simulink model "IEEE34bus_v2019b_Phasor_PI"  (R2019b)
settings: Solver=ode4  StartTime=0.0  StopTime=100  FixedStep=Ts  MaxStep=1e-4  RelTol=1e-4
InitFcn:
  | a=1; % Loading Factor
  | Ts=0.1;% For Delay Blocks in Voltage Regulator Controls
  | % phase to sequence conversion of RXB matrices
  | c=1*exp(sqrt(-1)*(120*pi/180));
  | T=[1 1 1;1 c*c c;1 c c*c];
  | Tinv=1/3*[1 1 1;1 c c*c;1 c*c c];
  | 
  | % Simulation data for the IEEE 34 Node Test Feeder model
  | mi2km = 1.60934;%  miles to km conversion
  | ft2km = 0.0003048; % feet to km conversion
  | ms2F = 1*1e-6/(2*pi*60);% microsiemens to Farads conversion
  | 
  | %% Configuration 300 - series reactance - ohm/mile
  | R_300 = [1.3368 0.2101 0.2130;0.2101 1.3238 0.2066;0.2130 0.2066 1.3294];
  | X_300 = [1.3343 0.5779 0.5015;0.5779 1.3569 0.4591;0.5015 0.4591 1.3471];
  | % charging susceptance - microsiemens/mile
  | B_300 = [5.3350 -1.5313 -0.9943;-1.5313 5.0979 -0.6212;-0.9943 -0.6212 4.8880];
  | 
  | R_300 = R_300/mi2km;
  | Rseq=Tinv*R_300*T;
  | R1_300=Rseq(2,2);R0_300=Rseq(1,1);
  | 
  | L_300 = (X_300/(2*pi*60))/mi2km;
  | Lseq=Tinv*L_300*T;
  | L1_300=Lseq(2,2);L0_300=Lseq(1,1);
  | 
  | C_300 =(B_300*ms2F)/mi2km;
  | Cseq=Tinv*C_300*T;
  | C1_300=Cseq(2,2);C0_300=Cseq(1,1);
  | 
  | %% Configuration 301 - series reactance - ohm/mile
  | R_301 = [1.9300 0.2327 0.2359;0.2327 1.9157 0.2288;0.2359 0.2288 1.9219];
  | X_301 = [1.4115 0.6442 0.5691;0.6442 1.4281 0.5238;0.5691 0.5238 1.4209];
  | % charging susceptance - microsiemens/mile
  | B_301 = [5.1207 -1.4364 -0.9402;-1.4364 4.9055 -0.5951;-0.9402 -0.5951 4.7154];
  | 
  | R_301 = R_301/mi2km;
  | Rseq=Tinv*R_301*T;
  | R1_301=Rseq(2,2);R0_301=Rseq(1,1);
  | 
  | L_301 = (X_301/(2*pi*60))/mi2km;
  | Lseq=Tinv*L_301*T;
  | L1_301=Lseq(2,2);L0_301=Lseq(1,1);
  | 
  | C_301 =(B_301*ms2F)/mi2km;
  | Cseq=Tinv*C_301*T;
  | C1_301=Cseq(2,2);C0_301=Cseq(1,1);
  | 
  | %% Configuration 302 - series reactance - ohm/mile
  | R_302 = [2.7995 0 0;0 0 0;0 0 0];
  | X_302 = [1.4855 0 0;0 0 0;0 0 0];
  | % charging susceptance - microsiemens/mile
  | B_302 = [4.2251 0 0;0 0 0;0 0 0];
  | 
  | R_302 = R_302/mi2km;
  | Rseq=Tinv*R_302*T;
  | R1_302=Rseq(2,2);R0_302=Rseq(1,1);
  | 
  | L_302 = (X_302/(2*pi*60))/mi2km;
  | Lseq=Tinv*L_302*T;
  | ... (+41 lines)
undefined symbols (not defined in the file or in its folder): find_system, j
libraries: powerlib x311, powerlib_meascontrol x22
(part 3 of 5)

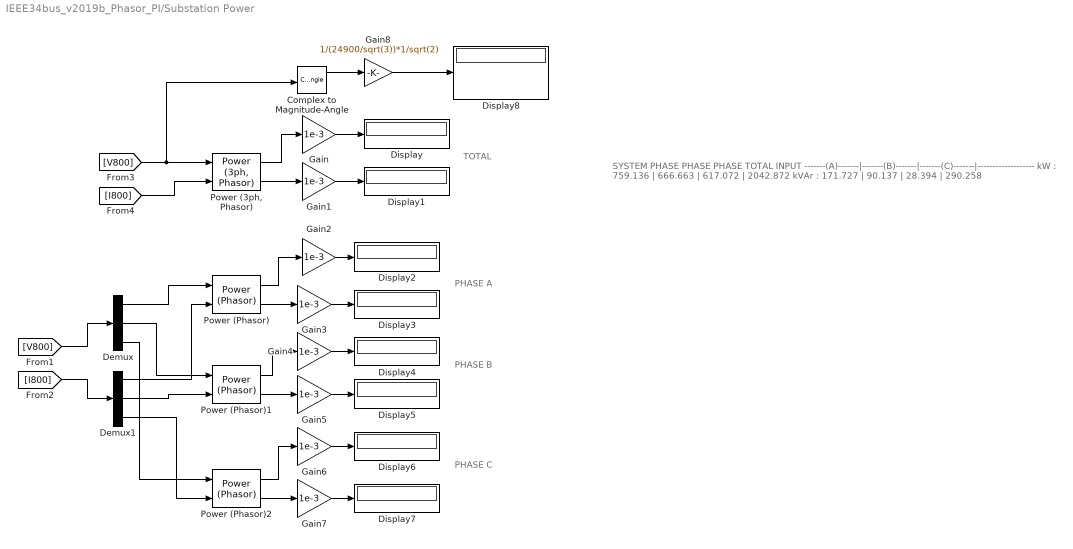
== system IEEE34bus_v2019b_Phasor_PI/Substation Power ==
  note: SYSTEM PHASE PHASE PHASE TOTAL
      | INPUT -------(A)-------|-------(B)-------|-------(C)-------|-------------------
      | kW : 759.136 | 666.663 | 617.072 | 2042.872
      | kVAr : 171.727 | 90.137 | 28.394 | 290.258
  note: PHASE C
  note: PHASE A
  note: PHASE B
  note: TOTAL
  Complex to Magnitude-Angle : ComplexToMagnitudeAngle
  Demux : Demux  Outputs=3
  Demux1 : Demux  Outputs=3
  Display{,1..8} (9 alike) : Display
  Gain{,1..7} (8 alike) : Gain  Gain=1e-3
  Gain8 : Gain  Gain=1/(24900/sqrt(3))*1/sqrt(2)
  "Power (3ph, Phasor)" : powerlib_meascontrol/Measurements/Power (3ph, Phasor)
      settings: SourceProductName=Simscape Electrical  SourceProductBaseCode=PS
  Power (Phasor) : powerlib_meascontrol/Measurements/Power (Phasor)
      settings: SourceProductName=Simscape Electrical  SourceProductBaseCode=PS
  Power (Phasor)1 : powerlib_meascontrol/Measurements/Power (Phasor)
      settings: SourceProductName=Simscape Electrical  SourceProductBaseCode=PS
  Power (Phasor)2 : powerlib_meascontrol/Measurements/Power (Phasor)
      settings: SourceProductName=Simscape Electrical  SourceProductBaseCode=PS
  wires:
  [I800] -> "Power (3ph, Phasor)"/2
  "Power (3ph, Phasor)"/1 -> Gain/1
  "Power (3ph, Phasor)"/2 -> Gain1/1
  [V800] -> Demux/1
  [I800] -> Demux1/1
  Demux/1 -> Power (Phasor)/1
  Demux1/1 -> Power (Phasor)/2
  Demux/2 -> Power (Phasor)1/1
  Demux1/2 -> Power (Phasor)1/2
  Demux/3 -> Power (Phasor)2/1
  Demux1/3 -> Power (Phasor)2/2
  Power (Phasor)/1 -> Gain2/1
  Power (Phasor)/2 -> Gain3/1
  Power (Phasor)1/1 -> Gain4/1
  Power (Phasor)1/2 -> Gain5/1
  Power (Phasor)2/1 -> Gain6/1
  Power (Phasor)2/2 -> Gain7/1
  Gain/1 -> Display/1
  Gain1/1 -> Display1/1
  Gain2/1 -> Display2/1
  Gain3/1 -> Display3/1
  Gain4/1 -> Display4/1
  Gain5/1 -> Display5/1
  Gain6/1 -> Display6/1
  Gain7/1 -> Display7/1
  Complex to Magnitude-Angle/1 -> Gain8/1
  [V800] -> Complex to Magnitude-Angle/1, "Power (3ph, Phasor)"/1
  Gain8/1 -> Display8/1

== system IEEE34bus_v2019b_Phasor_PI/Regulator 1/Single Phase SVR_A ==
  Line Drop Compensator : Subsystem
  Transformer with Taps : Subsystem
  Voltage Regulator Control : Subsystem
  S : PMIOPort  Tag=PMCPort  Side=Left
  L : PMIOPort  Tag=PMCPort  Port=2  Side=Right
  Tap : Outport  VectorParamsAs1DForOutWhenUnconnected=off
  tag scope: Vr1a=global
  wires:
  Line Drop Compensator/1(Vm) -> [Vr1a], Voltage Regulator Control/1(Vm)
  Voltage Regulator Control/1(Tap) -> Transformer with Taps/1(tap), Tap/1
  Transformer with Taps/1(Isec) -> Line Drop Compensator/1(Isec)
  Transformer with Taps/2(Vsec) -> Line Drop Compensator/2(Vsec)
  connections:
  Transformer with Taps/RConn1 -- L/RConn1
  Transformer with Taps/LConn1 -- S/RConn1

== system IEEE34bus_v2019b_Phasor_PI/Regulator 1/Single Phase SVR_B ==
  Line Drop Compensator : Subsystem
  Transformer with Taps : Subsystem
  Voltage Regulator Control : Subsystem
  S : PMIOPort  Tag=PMCPort  Side=Left
  L : PMIOPort  Tag=PMCPort  Port=2  Side=Right
  Tap : Outport  VectorParamsAs1DForOutWhenUnconnected=off
  tag scope: Vr1b=global
  wires:
  Transformer with Taps/2(Vsec) -> Line Drop Compensator/2(Vsec)
  Transformer with Taps/1(Isec) -> Line Drop Compensator/1(Isec)
  Voltage Regulator Control/1(Tap) -> Transformer with Taps/1(tap), Tap/1
  Line Drop Compensator/1(Vm) -> [Vr1b], Voltage Regulator Control/1(Vm)
  connections:
  Transformer with Taps/LConn1 -- S/RConn1
  Transformer with Taps/RConn1 -- L/RConn1

== system IEEE34bus_v2019b_Phasor_PI/Regulator 1/Single Phase SVR_C ==
  Line Drop Compensator : Subsystem
  Transformer with Taps : Subsystem
  Voltage Regulator Control : Subsystem
  S : PMIOPort  Tag=PMCPort  Side=Left
  L : PMIOPort  Tag=PMCPort  Port=2  Side=Right
  Tap : Outport  VectorParamsAs1DForOutWhenUnconnected=off
  tag scope: Vr1c=global
  wires:
  Line Drop Compensator/1(Vm) -> [Vr1c], Voltage Regulator Control/1(Vm)
  Voltage Regulator Control/1(Tap) -> Transformer with Taps/1(tap), Tap/1
  Transformer with Taps/1(Isec) -> Line Drop Compensator/1(Isec)
  Transformer with Taps/2(Vsec) -> Line Drop Compensator/2(Vsec)
  connections:
  Transformer with Taps/RConn1 -- L/RConn1
  Transformer with Taps/LConn1 -- S/RConn1

== system IEEE34bus_v2019b_Phasor_PI/Regulator 2/Single Phase SVR_A ==
  Line Drop Compensator : Subsystem
  Transformer with Taps : Subsystem
  Voltage Regulator Control : Subsystem
  S : PMIOPort  Tag=PMCPort  Side=Left
  L : PMIOPort  Tag=PMCPort  Port=2  Side=Right
  Tap : Outport  VectorParamsAs1DForOutWhenUnconnected=off
  tag scope: Vr2a=global
  wires:
  Line Drop Compensator/1(Vm) -> [Vr2a], Voltage Regulator Control/1(Vm)
  Voltage Regulator Control/1(Tap) -> Transformer with Taps/1(tap), Tap/1
  Transformer with Taps/1(Isec) -> Line Drop Compensator/1(Isec)
  Transformer with Taps/2(Vsec) -> Line Drop Compensator/2(Vsec)
  connections:
  Transformer with Taps/RConn1 -- L/RConn1
  Transformer with Taps/LConn1 -- S/RConn1

== system IEEE34bus_v2019b_Phasor_PI/Regulator 2/Single Phase SVR_B ==
  Line Drop Compensator : Subsystem
  Transformer with Taps : Subsystem
  Voltage Regulator Control : Subsystem
  S : PMIOPort  Tag=PMCPort  Side=Left
  L : PMIOPort  Tag=PMCPort  Port=2  Side=Right
  Tap : Outport  VectorParamsAs1DForOutWhenUnconnected=off
  tag scope: Vr2b=global
  wires:
  Transformer with Taps/2(Vsec) -> Line Drop Compensator/2(Vsec)
  Transformer with Taps/1(Isec) -> Line Drop Compensator/1(Isec)
  Voltage Regulator Control/1(Tap) -> Transformer with Taps/1(tap), Tap/1
  Line Drop Compensator/1(Vm) -> [Vr2b], Voltage Regulator Control/1(Vm)
  connections:
  Transformer with Taps/LConn1 -- S/RConn1
  Transformer with Taps/RConn1 -- L/RConn1

== system IEEE34bus_v2019b_Phasor_PI/Regulator 2/Single Phase SVR_C ==
  Line Drop Compensator : Subsystem
  Transformer with Taps : Subsystem
  Voltage Regulator Control : Subsystem
  S : PMIOPort  Tag=PMCPort  Side=Left
  L : PMIOPort  Tag=PMCPort  Port=2  Side=Right
  Tap : Outport  VectorParamsAs1DForOutWhenUnconnected=off
  tag scope: Vr2c=global
  wires:
  Line Drop Compensator/1(Vm) -> [Vr2c], Voltage Regulator Control/1(Vm)
  Voltage Regulator Control/1(Tap) -> Transformer with Taps/1(tap), Tap/1
  Transformer with Taps/1(Isec) -> Line Drop Compensator/1(Isec)
  Transformer with Taps/2(Vsec) -> Line Drop Compensator/2(Vsec)
  connections:
  Transformer with Taps/RConn1 -- L/RConn1
  Transformer with Taps/LConn1 -- S/RConn1

== system IEEE34bus_v2019b_Phasor_PI/Regulator 1/Single Phase SVR_A/Line Drop Compensator ==
  note: Vm=Vsec-Isec(Rc+jXc)
  Isec : Inport
  Vsec : Inport  Port=2
  Abs1 : Abs
  Gain4 : Gain  Gain=1/sqrt(2)
  Gain5 : Gain  Gain=Rc+j*Xc
  Gain6 : Gain  Gain=1/sqrt(2)
  Sum1 : Sum  Inputs=|+-
  Vm : Outport
  wires:
  Abs1/1 -> Vm/1
  Sum1/1 -> Abs1/1
  Isec/1 -> Gain4/1
  Vsec/1 -> Gain6/1
  Gain4/1 -> Gain5/1
  Gain6/1 -> Sum1/1
  Gain5/1 -> Sum1/2

== system IEEE34bus_v2019b_Phasor_PI/Regulator 1/Single Phase SVR_A/Transformer with Taps ==
  note: Isec on CT Ratio base
  note: Vsec on Pt Ratio base
  tap : Inport
  "    " : Gain  Gain=(1/ptRatio)
  " 1" : Gain  Gain=(1/ctRatio)
  CT : powerlib/Measurements/Current Measurement  PhasorSimulation=on  OutputType=Complex  PSBequivalent=0
      settings: SourceProductName=Simscape Electrical
  Ground1 : powerlib/Elements/Ground  LConnTagsString=a
      settings: SourceProductName=Simscape Electrical
  Ground2 : powerlib/Elements/Ground  LConnTagsString=a
      settings: SourceProductName=Simscape Electrical
  Ground3 : powerlib/Elements/Ground  LConnTagsString=a
      settings: SourceProductName=Simscape Electrical
  Memory : Memory
  Memory1 : Memory
  PT : powerlib/Measurements/Voltage Measurement  PhasorSimulation=on  OutputType=Complex  PSBequivalent=0
      settings: SourceProductName=Simscape Electrical
  Tap Changing Transformer : Subsystem  mask(Tap Changing Transformer){}
      mask help: Implements a Tap changing two-winding ideal transformer with taps at secondary.
      mask Display:
      | A=[-85 -45 -44 -34 -26 -21 -20 -22 -28 -37 -47 -57 -63 -63 -54 -44 -34 -26 -21 -20 -22 -28 -37 -47 -57 -63 -63 -54 -44 -34 -26 -21 -20 -22 -28 -37 -47 -57 -63 -63 -54 -44 -34 -26 -21 -20 -22 -28 -37 -45 -45 -85];
      | B=[-50 -50 -50 -49 -45 -39 -33 -26 -21 -18 -17 -19 -22 -22 -26 -27 -25 -22 -16 -9 -3 2 6 6 4 1 1 -3 -4 -2 2 7 14 20 26 29 30 28 24 24 21 20 21 25 31 37 44 49 50 50 50 50];
      | C=[85 45 44 34 26 21 20 22 28 37 47 57 63 75 63 54 44 34 26 21 20 22 28 37 47 57 63 75 63 54 44 34 26 21 20 22 28 37 47 57 63 75 63 54 44 34 26 21 20 22 28 37 45 45 85];
      | D=[-50 -50 -50 -49 -45 -39 -33 -26 -21 -18 -17 -19 -22 -22 -22 -26 -27 -25 -22 -16 -9 -3 2 6 6 4 1 1 1 -3 -4 -2 2 7 14 20 26 29 30 28 24 24 24 21 20 21 25 31 37 44 49 50 50 50 50];
      | plot(-85,-100,85,100,A,B,C,D);
      | text(-50,-70, '1');text(40,-70, '2');
      | color('green')
      | port_label('Lconn',1,'+');port_label('Rconn',1,'+');
      | color('blue')
      | disp('N')
  L : PMIOPort  Tag=PMCPort  Side=Right
  S : PMIOPort  Port=2  Side=Left
  Isec : Outport
  Vsec : Outport  Port=2
  wires:
  tap/1 -> Tap Changing Transformer/1(Tap)
  Memory/1 -> Isec/1
  Memory1/1 -> Vsec/1
  " 1"/1 -> Memory/1
  CT/1 -> " 1"/1
  PT/1 -> "    "/1
  "    "/1 -> Memory1/1
  connections:
  Tap Changing Transformer/LConn2 -- Ground3/LConn1
  Tap Changing Transformer/LConn1 -- S/RConn1
  Tap Changing Transformer/RConn2 -- Ground2/LConn1
  CT/RConn1 -- L/RConn1
  PT/LConn1 -- CT/LConn1 -- Tap Changing Transformer/RConn1
  PT/LConn2 -- Ground1/LConn1

== system IEEE34bus_v2019b_Phasor_PI/Regulator 1/Single Phase SVR_A/Voltage Regulator Control ==
  Vm : Inport
  Constant : Constant  Value=RegulatorOn
  Tap Changer Control : Subsystem  mask(Tap Changer Control){MinMaxTap=TapMinMax, InitialPosition=InitialTap, MecDelay=TapSelectionTime}
      mask prompts: MinMaxTap "Minimum and maximum tap number [ Min  Max ] :"; InitialPosition "Initial tap position"; MecDelay "Mechanical delay time"
      mask init:
      | if MecDelay<=0,
      | 	MecDelay=1/60;
      | end
  Voltage regulator : Subsystem  mask{Vref=RegulatorVref*120, DeadBand=RegulatorDeadBand*120, TimeDelay=RegulatorDelay}
      mask prompts: Vref "Vref (on 120v base)"; DeadBand "Deadband (on 120v base)"; TimeDelay "Time delay (s)"
  Tap : Outport
  wires:
  Voltage regulator/2(Down) -> Tap Changer Control/2("Down ")
  Tap Changer Control/1(TapNo) -> Tap/1  "Tap"
  Voltage regulator/1(Up) -> Tap Changer Control/1("Up ")
  Tap Changer Control/2(Ready) -> Voltage regulator/2(Ready)
  Constant/1 -> Voltage regulator/3(RegOn)
  Vm/1 -> Voltage regulator/1(Vmes (pu))

== system IEEE34bus_v2019b_Phasor_PI/Regulator 1/Single Phase SVR_B/Line Drop Compensator ==
  note: Vm=Vsec-Isec(Rc+jXc)
  Isec : Inport
  Vsec : Inport  Port=2
  Abs1 : Abs
  Gain4 : Gain  Gain=1/sqrt(2)
  Gain5 : Gain  Gain=Rc+j*Xc
  Gain6 : Gain  Gain=1/sqrt(2)
  Sum1 : Sum  Inputs=|+-
  Vm : Outport
  wires:
  Abs1/1 -> Vm/1
  Sum1/1 -> Abs1/1
  Isec/1 -> Gain4/1
  Vsec/1 -> Gain6/1
  Gain4/1 -> Gain5/1
  Gain6/1 -> Sum1/1
  Gain5/1 -> Sum1/2

== system IEEE34bus_v2019b_Phasor_PI/Regulator 1/Single Phase SVR_B/Transformer with Taps ==
  note: Isec on CT Ratio base
  note: Vsec on Pt Ratio base
  tap : Inport
  "    " : Gain  Gain=(1/ptRatio)
  " 1" : Gain  Gain=(1/ctRatio)
  CT : powerlib/Measurements/Current Measurement  PhasorSimulation=on  OutputType=Complex  PSBequivalent=0
      settings: SourceProductName=Simscape Electrical
  Ground1 : powerlib/Elements/Ground  LConnTagsString=a
      settings: SourceProductName=Simscape Electrical
  Ground2 : powerlib/Elements/Ground  LConnTagsString=a
      settings: SourceProductName=Simscape Electrical
  Ground3 : powerlib/Elements/Ground  LConnTagsString=a
      settings: SourceProductName=Simscape Electrical
  Memory : Memory
  Memory1 : Memory
  PT : powerlib/Measurements/Voltage Measurement  PhasorSimulation=on  OutputType=Complex  PSBequivalent=0
      settings: SourceProductName=Simscape Electrical
  Tap Changing Transformer : Subsystem  mask(Tap Changing Transformer){}
      mask help: Implements a Tap changing two-winding ideal transformer with taps at secondary.
      mask Display:
      | A=[-85 -45 -44 -34 -26 -21 -20 -22 -28 -37 -47 -57 -63 -63 -54 -44 -34 -26 -21 -20 -22 -28 -37 -47 -57 -63 -63 -54 -44 -34 -26 -21 -20 -22 -28 -37 -47 -57 -63 -63 -54 -44 -34 -26 -21 -20 -22 -28 -37 -45 -45 -85];
      | B=[-50 -50 -50 -49 -45 -39 -33 -26 -21 -18 -17 -19 -22 -22 -26 -27 -25 -22 -16 -9 -3 2 6 6 4 1 1 -3 -4 -2 2 7 14 20 26 29 30 28 24 24 21 20 21 25 31 37 44 49 50 50 50 50];
      | C=[85 45 44 34 26 21 20 22 28 37 47 57 63 75 63 54 44 34 26 21 20 22 28 37 47 57 63 75 63 54 44 34 26 21 20 22 28 37 47 57 63 75 63 54 44 34 26 21 20 22 28 37 45 45 85];
      | D=[-50 -50 -50 -49 -45 -39 -33 -26 -21 -18 -17 -19 -22 -22 -22 -26 -27 -25 -22 -16 -9 -3 2 6 6 4 1 1 1 -3 -4 -2 2 7 14 20 26 29 30 28 24 24 24 21 20 21 25 31 37 44 49 50 50 50 50];
      | plot(-85,-100,85,100,A,B,C,D);
      | text(-50,-70, '1');text(40,-70, '2');
      | color('green')
      | port_label('Lconn',1,'+');port_label('Rconn',1,'+');
      | color('blue')
      | disp('N')
  L : PMIOPort  Tag=PMCPort  Side=Right
  S : PMIOPort  Port=2  Side=Left
  Isec : Outport
  Vsec : Outport  Port=2
  wires:
  tap/1 -> Tap Changing Transformer/1(Tap)
  Memory/1 -> Isec/1
  Memory1/1 -> Vsec/1
  " 1"/1 -> Memory/1
  CT/1 -> " 1"/1
  PT/1 -> "    "/1
  "    "/1 -> Memory1/1
  connections:
  Tap Changing Transformer/LConn2 -- Ground3/LConn1
  Tap Changing Transformer/LConn1 -- S/RConn1
  Tap Changing Transformer/RConn2 -- Ground2/LConn1
  CT/RConn1 -- L/RConn1
  PT/LConn1 -- CT/LConn1 -- Tap Changing Transformer/RConn1
  PT/LConn2 -- Ground1/LConn1

== system IEEE34bus_v2019b_Phasor_PI/Regulator 1/Single Phase SVR_B/Voltage Regulator Control ==
  Vm : Inport
  Constant : Constant  Value=RegulatorOn
  Tap Changer Control : Subsystem  mask(Tap Changer Control){MinMaxTap=TapMinMax, InitialPosition=InitialTap, MecDelay=TapSelectionTime}
      mask prompts: MinMaxTap "Minimum and maximum tap number [ Min  Max ] :"; InitialPosition "Initial tap position"; MecDelay "Mechanical delay time"
      mask init:
      | if MecDelay<=0,
      | 	MecDelay=1/60;
      | end
  Voltage regulator : Subsystem  mask{Vref=RegulatorVref*120, DeadBand=RegulatorDeadBand*120, TimeDelay=RegulatorDelay}
      mask prompts: Vref "Vref (on 120v base)"; DeadBand "Deadband (on 120v base)"; TimeDelay "Time delay (s)"
  Tap : Outport
  wires:
  Voltage regulator/2(Down) -> Tap Changer Control/2("Down ")
  Tap Changer Control/1(TapNo) -> Tap/1  "Tap"
  Voltage regulator/1(Up) -> Tap Changer Control/1("Up ")
  Tap Changer Control/2(Ready) -> Voltage regulator/2(Ready)
  Constant/1 -> Voltage regulator/3(RegOn)
  Vm/1 -> Voltage regulator/1(Vmes (pu))

== system IEEE34bus_v2019b_Phasor_PI/Regulator 1/Single Phase SVR_C/Line Drop Compensator ==
  note: Vm=Vsec-Isec(Rc+jXc)
  Isec : Inport
  Vsec : Inport  Port=2
  Abs1 : Abs
  Gain4 : Gain  Gain=1/sqrt(2)
  Gain5 : Gain  Gain=Rc+j*Xc
  Gain6 : Gain  Gain=1/sqrt(2)
  Sum1 : Sum  Inputs=|+-
  Vm : Outport
  wires:
  Abs1/1 -> Vm/1
  Sum1/1 -> Abs1/1
  Isec/1 -> Gain4/1
  Vsec/1 -> Gain6/1
  Gain4/1 -> Gain5/1
  Gain6/1 -> Sum1/1
  Gain5/1 -> Sum1/2

== system IEEE34bus_v2019b_Phasor_PI/Regulator 1/Single Phase SVR_C/Transformer with Taps ==
  note: Isec on CT Ratio base
  note: Vsec on Pt Ratio base
  tap : Inport
  "    " : Gain  Gain=(1/ptRatio)
  " 1" : Gain  Gain=(1/ctRatio)
  CT : powerlib/Measurements/Current Measurement  PhasorSimulation=on  OutputType=Complex  PSBequivalent=0
      settings: SourceProductName=Simscape Electrical
  Ground1 : powerlib/Elements/Ground  LConnTagsString=a
      settings: SourceProductName=Simscape Electrical
  Ground2 : powerlib/Elements/Ground  LConnTagsString=a
      settings: SourceProductName=Simscape Electrical
  Ground3 : powerlib/Elements/Ground  LConnTagsString=a
      settings: SourceProductName=Simscape Electrical
  Memory : Memory
  Memory1 : Memory
  PT : powerlib/Measurements/Voltage Measurement  PhasorSimulation=on  OutputType=Complex  PSBequivalent=0
      settings: SourceProductName=Simscape Electrical
  Tap Changing Transformer : Subsystem  mask(Tap Changing Transformer){}
      mask help: Implements a Tap changing two-winding ideal transformer with taps at secondary.
      mask Display:
      | A=[-85 -45 -44 -34 -26 -21 -20 -22 -28 -37 -47 -57 -63 -63 -54 -44 -34 -26 -21 -20 -22 -28 -37 -47 -57 -63 -63 -54 -44 -34 -26 -21 -20 -22 -28 -37 -47 -57 -63 -63 -54 -44 -34 -26 -21 -20 -22 -28 -37 -45 -45 -85];
      | B=[-50 -50 -50 -49 -45 -39 -33 -26 -21 -18 -17 -19 -22 -22 -26 -27 -25 -22 -16 -9 -3 2 6 6 4 1 1 -3 -4 -2 2 7 14 20 26 29 30 28 24 24 21 20 21 25 31 37 44 49 50 50 50 50];
      | C=[85 45 44 34 26 21 20 22 28 37 47 57 63 75 63 54 44 34 26 21 20 22 28 37 47 57 63 75 63 54 44 34 26 21 20 22 28 37 47 57 63 75 63 54 44 34 26 21 20 22 28 37 45 45 85];
      | D=[-50 -50 -50 -49 -45 -39 -33 -26 -21 -18 -17 -19 -22 -22 -22 -26 -27 -25 -22 -16 -9 -3 2 6 6 4 1 1 1 -3 -4 -2 2 7 14 20 26 29 30 28 24 24 24 21 20 21 25 31 37 44 49 50 50 50 50];
      | plot(-85,-100,85,100,A,B,C,D);
      | text(-50,-70, '1');text(40,-70, '2');
      | color('green')
      | port_label('Lconn',1,'+');port_label('Rconn',1,'+');
      | color('blue')
      | disp('N')
  L : PMIOPort  Tag=PMCPort  Side=Right
  S : PMIOPort  Port=2  Side=Left
  Isec : Outport
  Vsec : Outport  Port=2
  wires:
  tap/1 -> Tap Changing Transformer/1(Tap)
  Memory/1 -> Isec/1
  Memory1/1 -> Vsec/1
  " 1"/1 -> Memory/1
  CT/1 -> " 1"/1
  PT/1 -> "    "/1
  "    "/1 -> Memory1/1
  connections:
  Tap Changing Transformer/LConn2 -- Ground3/LConn1
  Tap Changing Transformer/LConn1 -- S/RConn1
  Tap Changing Transformer/RConn2 -- Ground2/LConn1
  CT/RConn1 -- L/RConn1
  PT/LConn1 -- CT/LConn1 -- Tap Changing Transformer/RConn1
  PT/LConn2 -- Ground1/LConn1

== system IEEE34bus_v2019b_Phasor_PI/Regulator 1/Single Phase SVR_C/Voltage Regulator Control ==
  Vm : Inport
  Constant : Constant  Value=RegulatorOn
  Tap Changer Control : Subsystem  mask(Tap Changer Control){MinMaxTap=TapMinMax, InitialPosition=InitialTap, MecDelay=TapSelectionTime}
      mask prompts: MinMaxTap "Minimum and maximum tap number [ Min  Max ] :"; InitialPosition "Initial tap position"; MecDelay "Mechanical delay time"
      mask init:
      | if MecDelay<=0,
      | 	MecDelay=1/60;
      | end
  Voltage regulator : Subsystem  mask{Vref=RegulatorVref*120, DeadBand=RegulatorDeadBand*120, TimeDelay=RegulatorDelay}
      mask prompts: Vref "Vref (on 120v base)"; DeadBand "Deadband (on 120v base)"; TimeDelay "Time delay (s)"
  Tap : Outport
  wires:
  Voltage regulator/2(Down) -> Tap Changer Control/2("Down ")
  Tap Changer Control/1(TapNo) -> Tap/1  "Tap"
  Voltage regulator/1(Up) -> Tap Changer Control/1("Up ")
  Tap Changer Control/2(Ready) -> Voltage regulator/2(Ready)
  Constant/1 -> Voltage regulator/3(RegOn)
  Vm/1 -> Voltage regulator/1(Vmes (pu))

== system IEEE34bus_v2019b_Phasor_PI/Regulator 2/Single Phase SVR_A/Line Drop Compensator ==
  note: Vm=Vsec-Isec(Rc+jXc)
  Isec : Inport
  Vsec : Inport  Port=2
  Abs1 : Abs
  Gain4 : Gain  Gain=1/sqrt(2)
  Gain5 : Gain  Gain=Rc+j*Xc
  Gain6 : Gain  Gain=1/sqrt(2)
  Sum1 : Sum  Inputs=|+-
  Vm : Outport
  wires:
  Abs1/1 -> Vm/1
  Sum1/1 -> Abs1/1
  Isec/1 -> Gain4/1
  Vsec/1 -> Gain6/1
  Gain4/1 -> Gain5/1
  Gain6/1 -> Sum1/1
  Gain5/1 -> Sum1/2

== system IEEE34bus_v2019b_Phasor_PI/Regulator 2/Single Phase SVR_A/Transformer with Taps ==
  note: Isec on CT Ratio base
  note: Vsec on Pt Ratio base
  tap : Inport
  "    " : Gain  Gain=(1/ptRatio)
  " 1" : Gain  Gain=(1/ctRatio)
  CT : powerlib/Measurements/Current Measurement  PhasorSimulation=on  OutputType=Complex  PSBequivalent=0
      settings: SourceProductName=Simscape Electrical
  Ground1 : powerlib/Elements/Ground  LConnTagsString=a
      settings: SourceProductName=Simscape Electrical
  Ground2 : powerlib/Elements/Ground  LConnTagsString=a
      settings: SourceProductName=Simscape Electrical
  Ground3 : powerlib/Elements/Ground  LConnTagsString=a
      settings: SourceProductName=Simscape Electrical
  Memory : Memory
  Memory1 : Memory
  PT : powerlib/Measurements/Voltage Measurement  PhasorSimulation=on  OutputType=Complex  PSBequivalent=0
      settings: SourceProductName=Simscape Electrical
  Tap Changing Transformer : Subsystem  mask(Tap Changing Transformer){}
      mask help: Implements a Tap changing two-winding ideal transformer with taps at secondary.
      mask Display:
      | A=[-85 -45 -44 -34 -26 -21 -20 -22 -28 -37 -47 -57 -63 -63 -54 -44 -34 -26 -21 -20 -22 -28 -37 -47 -57 -63 -63 -54 -44 -34 -26 -21 -20 -22 -28 -37 -47 -57 -63 -63 -54 -44 -34 -26 -21 -20 -22 -28 -37 -45 -45 -85];
      | B=[-50 -50 -50 -49 -45 -39 -33 -26 -21 -18 -17 -19 -22 -22 -26 -27 -25 -22 -16 -9 -3 2 6 6 4 1 1 -3 -4 -2 2 7 14 20 26 29 30 28 24 24 21 20 21 25 31 37 44 49 50 50 50 50];
      | C=[85 45 44 34 26 21 20 22 28 37 47 57 63 75 63 54 44 34 26 21 20 22 28 37 47 57 63 75 63 54 44 34 26 21 20 22 28 37 47 57 63 75 63 54 44 34 26 21 20 22 28 37 45 45 85];
      | D=[-50 -50 -50 -49 -45 -39 -33 -26 -21 -18 -17 -19 -22 -22 -22 -26 -27 -25 -22 -16 -9 -3 2 6 6 4 1 1 1 -3 -4 -2 2 7 14 20 26 29 30 28 24 24 24 21 20 21 25 31 37 44 49 50 50 50 50];
      | plot(-85,-100,85,100,A,B,C,D);
      | text(-50,-70, '1');text(40,-70, '2');
      | color('green')
      | port_label('Lconn',1,'+');port_label('Rconn',1,'+');
      | color('blue')
      | disp('N')
  L : PMIOPort  Tag=PMCPort  Side=Right
  S : PMIOPort  Port=2  Side=Left
  Isec : Outport
  Vsec : Outport  Port=2
  wires:
  tap/1 -> Tap Changing Transformer/1(Tap)
  Memory/1 -> Isec/1
  Memory1/1 -> Vsec/1
  " 1"/1 -> Memory/1
  CT/1 -> " 1"/1
  PT/1 -> "    "/1
  "    "/1 -> Memory1/1
  connections:
  Tap Changing Transformer/LConn2 -- Ground3/LConn1
  Tap Changing Transformer/LConn1 -- S/RConn1
  Tap Changing Transformer/RConn2 -- Ground2/LConn1
  CT/RConn1 -- L/RConn1
  PT/LConn1 -- CT/LConn1 -- Tap Changing Transformer/RConn1
  PT/LConn2 -- Ground1/LConn1

== system IEEE34bus_v2019b_Phasor_PI/Regulator 2/Single Phase SVR_A/Voltage Regulator Control ==
  Vm : Inport
  Constant : Constant  Value=RegulatorOn
  Tap Changer Control : Subsystem  mask(Tap Changer Control){MinMaxTap=TapMinMax, InitialPosition=InitialTap, MecDelay=TapSelectionTime}
      mask prompts: MinMaxTap "Minimum and maximum tap number [ Min  Max ] :"; InitialPosition "Initial tap position"; MecDelay "Mechanical delay time"
      mask init:
      | if MecDelay<=0,
      | 	MecDelay=1/60;
      | end
  Voltage regulator : Subsystem  mask{Vref=RegulatorVref*120, DeadBand=RegulatorDeadBand*120, TimeDelay=RegulatorDelay}
      mask prompts: Vref "Vref (on 120v base)"; DeadBand "Deadband (on 120v base)"; TimeDelay "Time delay (s)"
  Tap : Outport
  wires:
  Voltage regulator/2(Down) -> Tap Changer Control/2("Down ")
  Tap Changer Control/1(TapNo) -> Tap/1  "Tap"
  Voltage regulator/1(Up) -> Tap Changer Control/1("Up ")
  Tap Changer Control/2(Ready) -> Voltage regulator/2(Ready)
  Constant/1 -> Voltage regulator/3(RegOn)
  Vm/1 -> Voltage regulator/1(Vmes (pu))

== system IEEE34bus_v2019b_Phasor_PI/Regulator 2/Single Phase SVR_B/Line Drop Compensator ==
  note: Vm=Vsec-Isec(Rc+jXc)
  Isec : Inport
  Vsec : Inport  Port=2
  Abs1 : Abs
  Gain4 : Gain  Gain=1/sqrt(2)
  Gain5 : Gain  Gain=Rc+j*Xc
  Gain6 : Gain  Gain=1/sqrt(2)
  Sum1 : Sum  Inputs=|+-
  Vm : Outport
  wires:
  Abs1/1 -> Vm/1
  Sum1/1 -> Abs1/1
  Isec/1 -> Gain4/1
  Vsec/1 -> Gain6/1
  Gain4/1 -> Gain5/1
  Gain6/1 -> Sum1/1
  Gain5/1 -> Sum1/2

== system IEEE34bus_v2019b_Phasor_PI/Regulator 2/Single Phase SVR_B/Transformer with Taps ==
  note: Isec on CT Ratio base
  note: Vsec on Pt Ratio base
  tap : Inport
  "    " : Gain  Gain=(1/ptRatio)
  " 1" : Gain  Gain=(1/ctRatio)
  CT : powerlib/Measurements/Current Measurement  PhasorSimulation=on  OutputType=Complex  PSBequivalent=0
      settings: SourceProductName=Simscape Electrical
  Ground1 : powerlib/Elements/Ground  LConnTagsString=a
      settings: SourceProductName=Simscape Electrical
  Ground2 : powerlib/Elements/Ground  LConnTagsString=a
      settings: SourceProductName=Simscape Electrical
  Ground3 : powerlib/Elements/Ground  LConnTagsString=a
      settings: SourceProductName=Simscape Electrical
  Memory : Memory
  Memory1 : Memory
  PT : powerlib/Measurements/Voltage Measurement  PhasorSimulation=on  OutputType=Complex  PSBequivalent=0
      settings: SourceProductName=Simscape Electrical
  Tap Changing Transformer : Subsystem  mask(Tap Changing Transformer){}
      mask help: Implements a Tap changing two-winding ideal transformer with taps at secondary.
      mask Display:
      | A=[-85 -45 -44 -34 -26 -21 -20 -22 -28 -37 -47 -57 -63 -63 -54 -44 -34 -26 -21 -20 -22 -28 -37 -47 -57 -63 -63 -54 -44 -34 -26 -21 -20 -22 -28 -37 -47 -57 -63 -63 -54 -44 -34 -26 -21 -20 -22 -28 -37 -45 -45 -85];
      | B=[-50 -50 -50 -49 -45 -39 -33 -26 -21 -18 -17 -19 -22 -22 -26 -27 -25 -22 -16 -9 -3 2 6 6 4 1 1 -3 -4 -2 2 7 14 20 26 29 30 28 24 24 21 20 21 25 31 37 44 49 50 50 50 50];
      | C=[85 45 44 34 26 21 20 22 28 37 47 57 63 75 63 54 44 34 26 21 20 22 28 37 47 57 63 75 63 54 44 34 26 21 20 22 28 37 47 57 63 75 63 54 44 34 26 21 20 22 28 37 45 45 85];
      | D=[-50 -50 -50 -49 -45 -39 -33 -26 -21 -18 -17 -19 -22 -22 -22 -26 -27 -25 -22 -16 -9 -3 2 6 6 4 1 1 1 -3 -4 -2 2 7 14 20 26 29 30 28 24 24 24 21 20 21 25 31 37 44 49 50 50 50 50];
      | plot(-85,-100,85,100,A,B,C,D);
      | text(-50,-70, '1');text(40,-70, '2');
      | color('green')
      | port_label('Lconn',1,'+');port_label('Rconn',1,'+');
      | color('blue')
      | disp('N')
  L : PMIOPort  Tag=PMCPort  Side=Right
  S : PMIOPort  Port=2  Side=Left
  Isec : Outport
  Vsec : Outport  Port=2
  wires:
  tap/1 -> Tap Changing Transformer/1(Tap)
  Memory/1 -> Isec/1
  Memory1/1 -> Vsec/1
  " 1"/1 -> Memory/1
  CT/1 -> " 1"/1
  PT/1 -> "    "/1
  "    "/1 -> Memory1/1
  connections:
  Tap Changing Transformer/LConn2 -- Ground3/LConn1
  Tap Changing Transformer/LConn1 -- S/RConn1
  Tap Changing Transformer/RConn2 -- Ground2/LConn1
  CT/RConn1 -- L/RConn1
  PT/LConn1 -- CT/LConn1 -- Tap Changing Transformer/RConn1
  PT/LConn2 -- Ground1/LConn1

== system IEEE34bus_v2019b_Phasor_PI/Regulator 2/Single Phase SVR_B/Voltage Regulator Control ==
  Vm : Inport
  Constant : Constant  Value=RegulatorOn
  Tap Changer Control : Subsystem  mask(Tap Changer Control){MinMaxTap=TapMinMax, InitialPosition=InitialTap, MecDelay=TapSelectionTime}
      mask prompts: MinMaxTap "Minimum and maximum tap number [ Min  Max ] :"; InitialPosition "Initial tap position"; MecDelay "Mechanical delay time"
      mask init:
      | if MecDelay<=0,
      | 	MecDelay=1/60;
      | end
  Voltage regulator : Subsystem  mask{Vref=RegulatorVref*120, DeadBand=RegulatorDeadBand*120, TimeDelay=RegulatorDelay}
      mask prompts: Vref "Vref (on 120v base)"; DeadBand "Deadband (on 120v base)"; TimeDelay "Time delay (s)"
  Tap : Outport
  wires:
  Voltage regulator/2(Down) -> Tap Changer Control/2("Down ")
  Tap Changer Control/1(TapNo) -> Tap/1  "Tap"
  Voltage regulator/1(Up) -> Tap Changer Control/1("Up ")
  Tap Changer Control/2(Ready) -> Voltage regulator/2(Ready)
  Constant/1 -> Voltage regulator/3(RegOn)
  Vm/1 -> Voltage regulator/1(Vmes (pu))

== system IEEE34bus_v2019b_Phasor_PI/Regulator 2/Single Phase SVR_C/Line Drop Compensator ==
  note: Vm=Vsec-Isec(Rc+jXc)
  Isec : Inport
  Vsec : Inport  Port=2
  Abs1 : Abs
  Gain4 : Gain  Gain=1/sqrt(2)
  Gain5 : Gain  Gain=Rc+j*Xc
  Gain6 : Gain  Gain=1/sqrt(2)
  Sum1 : Sum  Inputs=|+-
  Vm : Outport
  wires:
  Abs1/1 -> Vm/1
  Sum1/1 -> Abs1/1
  Isec/1 -> Gain4/1
  Vsec/1 -> Gain6/1
  Gain4/1 -> Gain5/1
  Gain6/1 -> Sum1/1
  Gain5/1 -> Sum1/2

== system IEEE34bus_v2019b_Phasor_PI/Regulator 2/Single Phase SVR_C/Transformer with Taps ==
  note: Isec on CT Ratio base
  note: Vsec on Pt Ratio base
  tap : Inport
  "    " : Gain  Gain=(1/ptRatio)
  " 1" : Gain  Gain=(1/ctRatio)
  CT : powerlib/Measurements/Current Measurement  PhasorSimulation=on  OutputType=Complex  PSBequivalent=0
      settings: SourceProductName=Simscape Electrical
  Ground1 : powerlib/Elements/Ground  LConnTagsString=a
      settings: SourceProductName=Simscape Electrical
  Ground2 : powerlib/Elements/Ground  LConnTagsString=a
      settings: SourceProductName=Simscape Electrical
  Ground3 : powerlib/Elements/Ground  LConnTagsString=a
      settings: SourceProductName=Simscape Electrical
  Memory : Memory
  Memory1 : Memory
  PT : powerlib/Measurements/Voltage Measurement  PhasorSimulation=on  OutputType=Complex  PSBequivalent=0
      settings: SourceProductName=Simscape Electrical
  Tap Changing Transformer : Subsystem  mask(Tap Changing Transformer){}
      mask help: Implements a Tap changing two-winding ideal transformer with taps at secondary.
      mask Display:
      | A=[-85 -45 -44 -34 -26 -21 -20 -22 -28 -37 -47 -57 -63 -63 -54 -44 -34 -26 -21 -20 -22 -28 -37 -47 -57 -63 -63 -54 -44 -34 -26 -21 -20 -22 -28 -37 -47 -57 -63 -63 -54 -44 -34 -26 -21 -20 -22 -28 -37 -45 -45 -85];
      | B=[-50 -50 -50 -49 -45 -39 -33 -26 -21 -18 -17 -19 -22 -22 -26 -27 -25 -22 -16 -9 -3 2 6 6 4 1 1 -3 -4 -2 2 7 14 20 26 29 30 28 24 24 21 20 21 25 31 37 44 49 50 50 50 50];
      | C=[85 45 44 34 26 21 20 22 28 37 47 57 63 75 63 54 44 34 26 21 20 22 28 37 47 57 63 75 63 54 44 34 26 21 20 22 28 37 47 57 63 75 63 54 44 34 26 21 20 22 28 37 45 45 85];
      | D=[-50 -50 -50 -49 -45 -39 -33 -26 -21 -18 -17 -19 -22 -22 -22 -26 -27 -25 -22 -16 -9 -3 2 6 6 4 1 1 1 -3 -4 -2 2 7 14 20 26 29 30 28 24 24 24 21 20 21 25 31 37 44 49 50 50 50 50];
      | plot(-85,-100,85,100,A,B,C,D);
      | text(-50,-70, '1');text(40,-70, '2');
      | color('green')
      | port_label('Lconn',1,'+');port_label('Rconn',1,'+');
      | color('blue')
      | disp('N')
  L : PMIOPort  Tag=PMCPort  Side=Right
  S : PMIOPort  Port=2  Side=Left
  Isec : Outport
  Vsec : Outport  Port=2
  wires:
  tap/1 -> Tap Changing Transformer/1(Tap)
  Memory/1 -> Isec/1
  Memory1/1 -> Vsec/1
  " 1"/1 -> Memory/1
  CT/1 -> " 1"/1
  PT/1 -> "    "/1
  "    "/1 -> Memory1/1
  connections:
  Tap Changing Transformer/LConn2 -- Ground3/LConn1
  Tap Changing Transformer/LConn1 -- S/RConn1
  Tap Changing Transformer/RConn2 -- Ground2/LConn1
  CT/RConn1 -- L/RConn1
  PT/LConn1 -- CT/LConn1 -- Tap Changing Transformer/RConn1
  PT/LConn2 -- Ground1/LConn1

== system IEEE34bus_v2019b_Phasor_PI/Regulator 2/Single Phase SVR_C/Voltage Regulator Control ==
  Vm : Inport
  Constant : Constant  Value=RegulatorOn
  Tap Changer Control : Subsystem  mask(Tap Changer Control){MinMaxTap=TapMinMax, InitialPosition=InitialTap, MecDelay=TapSelectionTime}
      mask prompts: MinMaxTap "Minimum and maximum tap number [ Min  Max ] :"; InitialPosition "Initial tap position"; MecDelay "Mechanical delay time"
      mask init:
      | if MecDelay<=0,
      | 	MecDelay=1/60;
      | end
  Voltage regulator : Subsystem  mask{Vref=RegulatorVref*120, DeadBand=RegulatorDeadBand*120, TimeDelay=RegulatorDelay}
      mask prompts: Vref "Vref (on 120v base)"; DeadBand "Deadband (on 120v base)"; TimeDelay "Time delay (s)"
  Tap : Outport
  wires:
  Voltage regulator/2(Down) -> Tap Changer Control/2("Down ")
  Tap Changer Control/1(TapNo) -> Tap/1  "Tap"
  Voltage regulator/1(Up) -> Tap Changer Control/1("Up ")
  Tap Changer Control/2(Ready) -> Voltage regulator/2(Ready)
  Constant/1 -> Voltage regulator/3(RegOn)
  Vm/1 -> Voltage regulator/1(Vmes (pu))

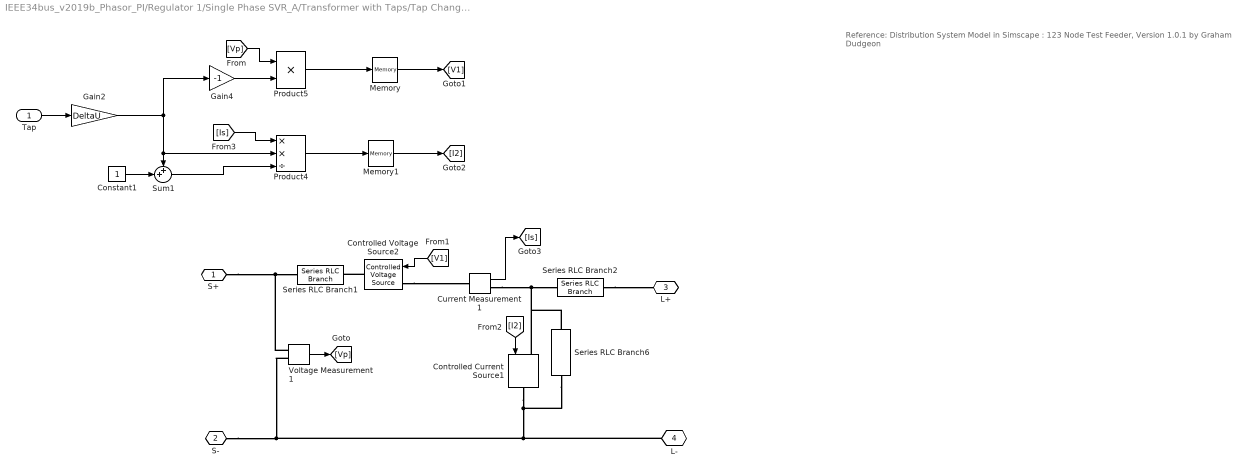
== system IEEE34bus_v2019b_Phasor_PI/Regulator 1/Single Phase SVR_A/Transformer with Taps/Tap Changing Transformer ==
  note: Reference:
      | Distribution System Model in Simscape : 123 Node Test Feeder, Version 1.0.1  by Graham Dudgeon
  Tap : Inport
  Constant1 : Constant
  Controlled Current Source1 : powerlib/Electrical Sources/Controlled Current Source  Initialize=off  Source_Type=AC  Amplitude=0  Phase=0  Frequency=0  Measurements=None
      settings: SourceProductName=Simscape Electrical
  Controlled Voltage Source2 : powerlib/Electrical Sources/Controlled Voltage Source  Initialize=off  Source_Type=AC  Amplitude=0  Phase=0  Frequency=0  Measurements=None
      settings: SourceProductName=Simscape Electrical
  Current Measurement1 : powerlib/Measurements/Current Measurement  PhasorSimulation=on  OutputType=Complex  PSBequivalent=0
      settings: SourceProductName=Simscape Electrical
  Gain2 : Gain  Gain=DeltaU
  Gain4 : Gain  Gain=-1
  Memory : Memory
  Memory1 : Memory
  Product4 : Product  Inputs=**/  RndMeth=Zero
  Product5 : Product  Inputs=**  RndMeth=Zero
  Series RLC Branch1 : powerlib/Elements/Series RLC Branch  LConnTagsString=__new0  RConnTagsString=__new0  BranchType=R  Resistance=1e-6  Inductance=1e-3  SetiL0=off  InitialCurrent=0  Capacitance=1e-6  Setx0=off  InitialVoltage=0  Measurements=None
      settings: SourceProductName=Simscape Electrical
  Series RLC Branch2 : powerlib/Elements/Series RLC Branch  LConnTagsString=__new0  RConnTagsString=__new0  BranchType=R  Resistance=1e-6  Inductance=1e-3  SetiL0=off  InitialCurrent=0  Capacitance=1e-6  Setx0=off  InitialVoltage=0  Measurements=None
      settings: SourceProductName=Simscape Electrical
  Series RLC Branch6 : powerlib/Elements/Series RLC Branch  LConnTagsString=__new0  RConnTagsString=__new0  BranchType=R  Resistance=1e6  Inductance=1e-3  SetiL0=off  InitialCurrent=0  Capacitance=1e-6  Setx0=off  InitialVoltage=0  Measurements=None
      settings: SourceProductName=Simscape Electrical
  Sum1 : Sum  Inputs=++|
  Voltage Measurement1 : powerlib/Measurements/Voltage Measurement  PhasorSimulation=on  OutputType=Complex  PSBequivalent=0
      settings: SourceProductName=Simscape Electrical
  S+ : PMIOPort  Side=Left
  S- : PMIOPort  Port=2  Side=Left
  L+ : PMIOPort  Port=3  Side=Right
  L- : PMIOPort  Port=4  Side=Right
  wires:
  Sum1/1 -> Product4/3
  [I2] -> Controlled Current Source1/1
  [V1] -> Controlled Voltage Source2/1
  Constant1/1 -> Sum1/2
  Product5/1 -> Memory/1
  Product4/1 -> Memory1/1
  [Is] -> Product4/1
  Current Measurement1/1 -> [Is]
  Tap/1 -> Gain2/1
  Gain2/1 -> Sum1/1, Product4/2, Gain4/1
  Gain4/1 -> Product5/2
  [Vp] -> Product5/1
  Voltage Measurement1/1 -> [Vp]
  Memory/1 -> [V1]
  Memory1/1 -> [I2]
  connections:
  Series RLC Branch6/LConn1 -- Controlled Current Source1/RConn1 -- S-/RConn1 -- Voltage Measurement1/LConn2 -- L-/RConn1
  Controlled Voltage Source2/RConn1 -- Series RLC Branch1/LConn1
  Current Measurement1/RConn1 -- Series RLC Branch6/RConn1 -- Controlled Current Source1/LConn1 -- Series RLC Branch2/RConn1
  Controlled Voltage Source2/LConn1 -- Current Measurement1/LConn1
  Voltage Measurement1/LConn1 -- Series RLC Branch1/RConn1 -- S+/RConn1
  Series RLC Branch2/LConn1 -- L+/RConn1

== system IEEE34bus_v2019b_Phasor_PI/Regulator 1/Single Phase SVR_A/Voltage Regulator Control/Tap Changer Control ==
  "Up " : Inport
  "Down " : Inport  Port=2
  Constant : Constant  Value=-1
  Constant1 : Constant
  Determine tap position : Subsystem
  Edge Detector : Subsystem  DialogController=POWERSYS.PowerSysDialog  mask(Edge Detector){model=Rising, ic=0}
      mask prompts: model "Edge:"; ic "Input at t = -eps:"
      mask help:
      | This block compares its present input to its previous input.
      |
      | If the input  is a logic signal (TRUE (1) or FALSE (0), the output is a one-step boolean signal TRUE  when  the specified edge (Rising, Falling or Either)  is detected.
      |
      | This block can also be used to detect the slope polarity of a continuous signal. For example, if the specified edge is  "Rising", the output is TRUE as long as the slope of the input signal is positive.
      |
      | The input value at time preceding t=0 is specified by the parameter "Input at t=-eps"
      mask init:
      | if model~=3,
      | 	x1 = (model -1)*20;
      |     x2 = (model -1)*60;
      | 	X1=[5,20,20,35]+25; Y1=[20+x2,20+x2,80-x2,80-x2];
      | 	X2=[5,20,35]+25;    Y2=[40+x1,60-x1,40+x1];
      | 	X3=[];X4=[];Y3=[];Y4=[];
      | else
      | 	x1 = 20;
      | 	x2 = 60;
      | 	X1=[5,20,20,35]+8; Y1=[20,20,80,80];
      | 	X2=[5,20,35]+8;    Y2=[40,60,40];
      | 	X3=[5,20,20,35]+53; Y3=[20+x2,20+x2,80-x2,80-x2];
      | 	X4=[5,20,35]+53;    Y4=[40+x1,60-x1,40+x1];
      | end
      | power_initmask();
      mask Help: This block is part of a subset of blocks in the Extras library that does not have documentation associated with it, other than the block mask description.
      mask TypeOptions model: Rising | Falling | Either
      mask Display: plot(0,0,100,100, X1,Y1,X2,Y2,X3,Y3,X4,Y4);
  Logical Operator : Logic  Operator=OR  AllPortsSameDT=off
  Logical Operator1 : Logic  AllPortsSameDT=off
  Mechanical Delay : TransportDelay  DelayTime=MecDelay  InitialOutput=InitialPosition  BufferSize=5120
  Memory : Memory  InitialCondition=1  InheritSampleTime=on
  Relational Operator : RelationalOperator  Operator===  OutDataTypeStr=float('double')  RndMeth=Nearest
  Switch : Switch  Threshold=0.5  SaturateOnIntegerOverflow=on
  TapNo : Outport  VectorParamsAs1DForOutWhenUnconnected=off
  Ready : Outport  Port=2  VectorParamsAs1DForOutWhenUnconnected=off
  wires:
  Mechanical Delay/1 -> TapNo/1, Relational Operator/2
  Logical Operator1/1 -> Determine tap position/Trigger
  "Up "/1 -> Logical Operator/1
  "Down "/1 -> Logical Operator/2, Switch/2
  Constant/1 -> Switch/1
  Constant1/1 -> Switch/3
  Switch/1 -> Determine tap position/1(NewTap)
  Determine tap position/1(TapNo) -> Mechanical Delay/1, Relational Operator/1
  Relational Operator/1 -> Memory/1
  Memory/1 -> Logical Operator1/1, Ready/1
  Logical Operator/1 -> Edge Detector/1(In)
  Edge Detector/1(Out) -> Logical Operator1/2

== system IEEE34bus_v2019b_Phasor_PI/Regulator 1/Single Phase SVR_A/Voltage Regulator Control/Voltage regulator ==
  Vmes (pu) : Inport
  Ready : Inport  Port=2
  RegOn : Inport  Port=3
  Dead Zone : DeadZone  LowerValue=-DeadBand/2  UpperValue=+DeadBand/2  SaturateOnIntegerOverflow=on
  Discrete Variable Time Delay : powerlib_meascontrol/Additional Components/Discrete Variable Time Delay  MaxDelay=3/60+Ts  InitialValue=1  Ts=Ts  DFT=on
      settings: SourceProductName=Simscape Electrical  SourceProductBaseCode=PS
  Logical Operator : Logic  AllPortsSameDT=off
  Logical Operator1 : Logic  AllPortsSameDT=off
  On Delay : powerlib_meascontrol/Logic/On Delay  DelayType=On delay  delay=TimeDelay  ic=0  Ts=Ts
      settings: SourceProductName=Simscape Electrical
  On Delay1 : powerlib_meascontrol/Logic/On Delay  DelayType=On delay  delay=TimeDelay  ic=0  Ts=Ts
      settings: SourceProductName=Simscape Electrical
  Relational Operator : RelationalOperator  Operator=>  RndMeth=Nearest
  Relational Operator1 : RelationalOperator  Operator=<  RndMeth=Nearest
  Sum : Sum  Inputs=|+-  SaturateOnIntegerOverflow=on
  Switch : Switch  Threshold=1.5  SaturateOnIntegerOverflow=on
  Vref : Constant  Value=Vref
  Vref1 : Constant  Value=0
  Vref2 : Constant  Value=0
  Vref3 : Constant  Value=0
  Vref4 : Constant  Value=3/60
  Up : Outport  VectorParamsAs1DForOutWhenUnconnected=off
  Down : Outport  Port=2  VectorParamsAs1DForOutWhenUnconnected=off
  wires:
  Vref2/1 -> Switch/3
  RegOn/1 -> Switch/2
  Switch/1 -> Dead Zone/1
  Sum/1 -> Switch/1
  Vref/1 -> Sum/1
  Vmes (pu)/1 -> Sum/2
  Dead Zone/1 -> Relational Operator1/1, Relational Operator/1
  Vref1/1 -> Relational Operator/2
  Relational Operator/1 -> Logical Operator/1
  Ready/1 -> Discrete Variable Time Delay/1
  Logical Operator/1 -> On Delay/1
  On Delay/1 -> Up/1
  Relational Operator1/1 -> Logical Operator1/2
  Logical Operator1/1 -> On Delay1/1
  On Delay1/1 -> Down/1
  Vref3/1 -> Relational Operator1/2
  Discrete Variable Time Delay/1 -> Logical Operator1/1, Logical Operator/2
  Vref4/1 -> Discrete Variable Time Delay/2

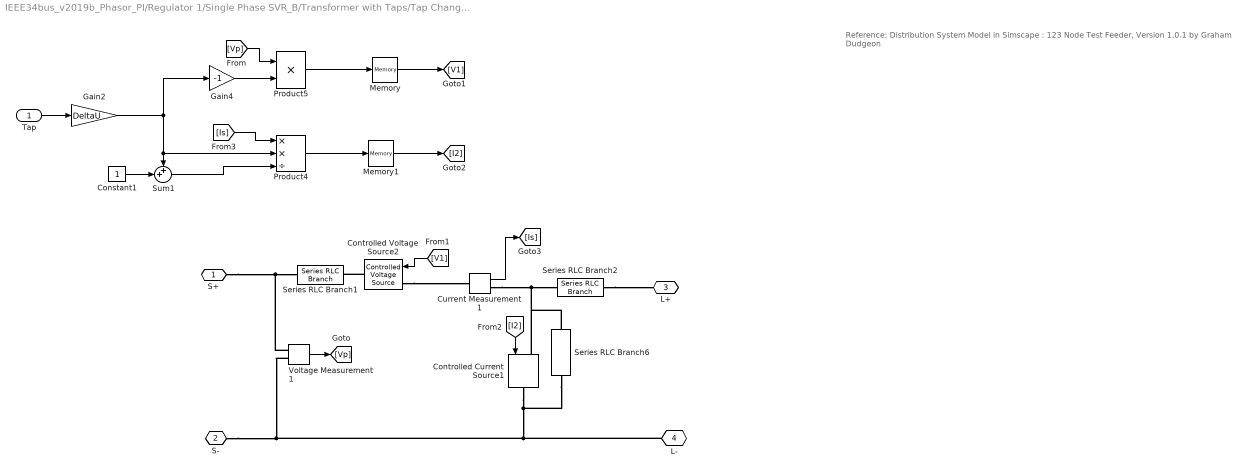
== system IEEE34bus_v2019b_Phasor_PI/Regulator 1/Single Phase SVR_B/Transformer with Taps/Tap Changing Transformer ==
  note: Reference:
      | Distribution System Model in Simscape : 123 Node Test Feeder, Version 1.0.1  by Graham Dudgeon
  Tap : Inport
  Constant1 : Constant
  Controlled Current Source1 : powerlib/Electrical Sources/Controlled Current Source  Initialize=off  Source_Type=AC  Amplitude=0  Phase=0  Frequency=0  Measurements=None
      settings: SourceProductName=Simscape Electrical
  Controlled Voltage Source2 : powerlib/Electrical Sources/Controlled Voltage Source  Initialize=off  Source_Type=AC  Amplitude=0  Phase=0  Frequency=0  Measurements=None
      settings: SourceProductName=Simscape Electrical
  Current Measurement1 : powerlib/Measurements/Current Measurement  PhasorSimulation=on  OutputType=Complex  PSBequivalent=0
      settings: SourceProductName=Simscape Electrical
  Gain2 : Gain  Gain=DeltaU
  Gain4 : Gain  Gain=-1
  Memory : Memory
  Memory1 : Memory
  Product4 : Product  Inputs=**/  RndMeth=Zero
  Product5 : Product  Inputs=**  RndMeth=Zero
  Series RLC Branch1 : powerlib/Elements/Series RLC Branch  LConnTagsString=__new0  RConnTagsString=__new0  BranchType=R  Resistance=1e-6  Inductance=1e-3  SetiL0=off  InitialCurrent=0  Capacitance=1e-6  Setx0=off  InitialVoltage=0  Measurements=None
      settings: SourceProductName=Simscape Electrical
  Series RLC Branch2 : powerlib/Elements/Series RLC Branch  LConnTagsString=__new0  RConnTagsString=__new0  BranchType=R  Resistance=1e-6  Inductance=1e-3  SetiL0=off  InitialCurrent=0  Capacitance=1e-6  Setx0=off  InitialVoltage=0  Measurements=None
      settings: SourceProductName=Simscape Electrical
  Series RLC Branch6 : powerlib/Elements/Series RLC Branch  LConnTagsString=__new0  RConnTagsString=__new0  BranchType=R  Resistance=1e6  Inductance=1e-3  SetiL0=off  InitialCurrent=0  Capacitance=1e-6  Setx0=off  InitialVoltage=0  Measurements=None
      settings: SourceProductName=Simscape Electrical
  Sum1 : Sum  Inputs=++|
  Voltage Measurement1 : powerlib/Measurements/Voltage Measurement  PhasorSimulation=on  OutputType=Complex  PSBequivalent=0
      settings: SourceProductName=Simscape Electrical
  S+ : PMIOPort  Side=Left
  S- : PMIOPort  Port=2  Side=Left
  L+ : PMIOPort  Port=3  Side=Right
  L- : PMIOPort  Port=4  Side=Right
  wires:
  Sum1/1 -> Product4/3
  [I2] -> Controlled Current Source1/1
  [V1] -> Controlled Voltage Source2/1
  Constant1/1 -> Sum1/2
  Product5/1 -> Memory/1
  Product4/1 -> Memory1/1
  [Is] -> Product4/1
  Current Measurement1/1 -> [Is]
  Tap/1 -> Gain2/1
  Gain2/1 -> Sum1/1, Product4/2, Gain4/1
  Gain4/1 -> Product5/2
  [Vp] -> Product5/1
  Voltage Measurement1/1 -> [Vp]
  Memory/1 -> [V1]
  Memory1/1 -> [I2]
  connections:
  Series RLC Branch6/LConn1 -- Controlled Current Source1/RConn1 -- S-/RConn1 -- Voltage Measurement1/LConn2 -- L-/RConn1
  Controlled Voltage Source2/RConn1 -- Series RLC Branch1/LConn1
  Current Measurement1/RConn1 -- Series RLC Branch6/RConn1 -- Controlled Current Source1/LConn1 -- Series RLC Branch2/RConn1
  Controlled Voltage Source2/LConn1 -- Current Measurement1/LConn1
  Voltage Measurement1/LConn1 -- Series RLC Branch1/RConn1 -- S+/RConn1
  Series RLC Branch2/LConn1 -- L+/RConn1

== system IEEE34bus_v2019b_Phasor_PI/Regulator 1/Single Phase SVR_B/Voltage Regulator Control/Tap Changer Control ==
  "Up " : Inport
  "Down " : Inport  Port=2
  Constant : Constant  Value=-1
  Constant1 : Constant
  Determine tap position : Subsystem
  Edge Detector : Subsystem  DialogController=POWERSYS.PowerSysDialog  mask(Edge Detector){model=Rising, ic=0}
      mask prompts: model "Edge:"; ic "Input at t = -eps:"
      mask help:
      | This block compares its present input to its previous input.
      |
      | If the input  is a logic signal (TRUE (1) or FALSE (0), the output is a one-step boolean signal TRUE  when  the specified edge (Rising, Falling or Either)  is detected.
      |
      | This block can also be used to detect the slope polarity of a continuous signal. For example, if the specified edge is  "Rising", the output is TRUE as long as the slope of the input signal is positive.
      |
      | The input value at time preceding t=0 is specified by the parameter "Input at t=-eps"
      mask init: same as IEEE34bus_v2019b_Phasor_PI/Regulator 1/Single Phase SVR_A/Voltage Regulator Control/Tap Changer Control/Edge Detector
      mask Help: This block is part of a subset of blocks in the Extras library that does not have documentation associated with it, other than the block mask description.
      mask TypeOptions model: Rising | Falling | Either
      mask Display: plot(0,0,100,100, X1,Y1,X2,Y2,X3,Y3,X4,Y4);
  Logical Operator : Logic  Operator=OR  AllPortsSameDT=off
  Logical Operator1 : Logic  AllPortsSameDT=off
  Mechanical Delay : TransportDelay  DelayTime=MecDelay  InitialOutput=InitialPosition  BufferSize=5120
  Memory : Memory  InitialCondition=1  InheritSampleTime=on
  Relational Operator : RelationalOperator  Operator===  OutDataTypeStr=float('double')  RndMeth=Nearest
  Switch : Switch  Threshold=0.5  SaturateOnIntegerOverflow=on
  TapNo : Outport  VectorParamsAs1DForOutWhenUnconnected=off
  Ready : Outport  Port=2  VectorParamsAs1DForOutWhenUnconnected=off
  wires:
  Mechanical Delay/1 -> TapNo/1, Relational Operator/2
  Logical Operator1/1 -> Determine tap position/Trigger
  "Up "/1 -> Logical Operator/1
  "Down "/1 -> Logical Operator/2, Switch/2
  Constant/1 -> Switch/1
  Constant1/1 -> Switch/3
  Switch/1 -> Determine tap position/1(NewTap)
  Determine tap position/1(TapNo) -> Mechanical Delay/1, Relational Operator/1
  Relational Operator/1 -> Memory/1
  Memory/1 -> Logical Operator1/1, Ready/1
  Logical Operator/1 -> Edge Detector/1(In)
  Edge Detector/1(Out) -> Logical Operator1/2
